simulink model "rm_rdm_2"  (Simulink 8.7)
settings: Solver=VariableStepAuto  StartTime=0.0  StopTime=30.0  RelTol=1e-3
settings Model: Creator=admin  LastModifiedBy=admin
settings DataIOCC: LimitDataPoints=off  SaveFormat=Dataset
settings DebuggingCC: UnderspecifiedInitializationDetection=Simplified  MergeDetectMultiDrivingBlocksExec=error
settings HardwareCC: ProdBitPerPointer=64  ProdLargestAtomicFloat=Float  ProdIntDivRoundTo=Zero  ProdEndianess=LittleEndian  ProdWordSize=64  ProdHWDeviceType=Intel->x86-64 (Windows64)
settings ModelReferenceCC: PropagateSignalLabelsOutOfModel=on
settings ConfigComp: CovModelRefEnable=off

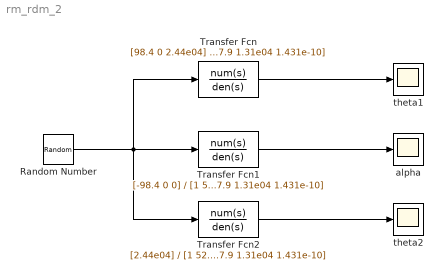
== system rm_rdm_2 ==
  Random Number : RandomNumber  SampleTime=0.1
  Transfer Fcn : TransferFcn  Numerator=[98.4 0 2.44e04]  Denominator=[1 52.84 947.9 1.31e04 1.431e-10]
  Transfer Fcn1 : TransferFcn  Numerator=[-98.4 0 0]  Denominator=[1 52.84 947.9 1.31e04 1.431e-10]
  Transfer Fcn2 : TransferFcn  Numerator=[2.44e04]  Denominator=[1 52.84 947.9 1.31e04 1.431e-10]
  alpha : Scope
  theta1 : Scope
  theta2 : Scope
  wires:
  Random Number/1 -> Transfer Fcn2/1, Transfer Fcn/1, Transfer Fcn1/1
  Transfer Fcn1/1 -> alpha/1
  Transfer Fcn/1 -> theta1/1
  Transfer Fcn2/1 -> theta2/1
